simulink model "PC_Quadcopter_Simulation_Alchemist"  (R2023b)
settings: Solver=ode4  StartTime=0  StopTime=Tf  FixedStep=Ts  MaxStep=0.06  RelTol=1e-3  EnableMultiTasking=on
model workspace (MAT data in the model file):
  Sig = Simulink.Signal
  Sig.DataType = 'auto'
  Sig.Dimensions = -1
  Sig.DimensionsMode = 'auto'
  Sig.Complexity = 'auto'
  Sig.SampleTime = -1
  Sig.SamplingMode = 'auto'
values from neighbouring files (symbols this model uses):
  den_Pphi = conv(den_Qphi, num_Gphi)    [PC_Quadcopter_Alchemist_woDOBC.m]    (also in workingOcto.m)
  den_Ppsi = conv(den_Qpsi, num_Gpsi)    [PC_Quadcopter_Alchemist_woDOBC.m]    (also in workingOcto.m)
  den_Ptheta = conv(den_Qtheta, num_Gtheta)    [PC_Quadcopter_Alchemist_woDOBC.m]    (also in workingOcto.m)
  den_Px = conv(den_Qx, num_Gx)    [PC_Quadcopter_Alchemist_woDOBC.m]    (also in workingOcto.m)
  den_Py = conv(den_Qy, num_Gy)    [PC_Quadcopter_Alchemist_woDOBC.m]    (also in workingOcto.m)
  den_Pz = conv(den_Qz, num_Gz)    [PC_Quadcopter_Alchemist_woDOBC.m]    (also in workingOcto.m)
  Dist_Amp_phi = 0    [PC_Quadcopter_Alchemist_woDOBC.m]    (also in workingOcto.m)
  Dist_Amp_psi = 0    [PC_Quadcopter_Alchemist_woDOBC.m]    (also in workingOcto.m)
  Dist_Amp_theta = 0    [PC_Quadcopter_Alchemist_woDOBC.m]    (also in workingOcto.m)
  Dist_Amp_x = 0    [PC_Quadcopter_Alchemist_woDOBC.m]    (also in workingOcto.m)
  Dist_Amp_y = 0    [PC_Quadcopter_Alchemist_woDOBC.m]    (also in workingOcto.m)
  Dist_Amp_z = 0    [PC_Quadcopter_Alchemist_woDOBC.m]    (also in workingOcto.m)
  Dist_Freq_phi = 0    [PC_Quadcopter_Alchemist_woDOBC.m]    (also in workingOcto.m)
  Dist_Freq_psi = 0    [PC_Quadcopter_Alchemist_woDOBC.m]    (also in workingOcto.m)
  Dist_Freq_theta = 0    [PC_Quadcopter_Alchemist_woDOBC.m]    (also in workingOcto.m)
  Dist_Freq_x = 0    [PC_Quadcopter_Alchemist_woDOBC.m]    (also in workingOcto.m)
  Dist_Freq_y = 0    [PC_Quadcopter_Alchemist_woDOBC.m]    (also in workingOcto.m)
  Dist_Freq_z = 0    [PC_Quadcopter_Alchemist_woDOBC.m]    (also in workingOcto.m)
  Dist_mean_phi = 0    [PC_Quadcopter_Alchemist_woDOBC.m]    (also in workingOcto.m)
  Dist_mean_psi = 0    [PC_Quadcopter_Alchemist_woDOBC.m]    (also in workingOcto.m)
  Dist_mean_theta = 0    [PC_Quadcopter_Alchemist_woDOBC.m]    (also in workingOcto.m)
  Dist_mean_x = 0    [PC_Quadcopter_Alchemist_woDOBC.m]    (also in workingOcto.m)
  Dist_mean_y = 0    [PC_Quadcopter_Alchemist_woDOBC.m]    (also in workingOcto.m)
  Dist_mean_z = 0    [PC_Quadcopter_Alchemist_woDOBC.m]    (also in workingOcto.m)
  Dist_Var_phi = 0    [PC_Quadcopter_Alchemist_woDOBC.m]    (also in workingOcto.m)
  Dist_Var_psi = 0    [PC_Quadcopter_Alchemist_woDOBC.m]    (also in workingOcto.m)
  Dist_Var_theta = 0    [PC_Quadcopter_Alchemist_woDOBC.m]    (also in workingOcto.m)
  Dist_Var_x = 0    [PC_Quadcopter_Alchemist_woDOBC.m]    (also in workingOcto.m)
  Dist_Var_y = 0    [PC_Quadcopter_Alchemist_woDOBC.m]    (also in workingOcto.m)
  Dist_Var_z = 0    [PC_Quadcopter_Alchemist_woDOBC.m]    (also in workingOcto.m)
  DISTURBANCE = 0    [PC_Quadcopter_Alchemist_woDOBC.m]    (also in workingOcto.m)
  DOBC_phi = 0    [PC_Quadcopter_Alchemist_woDOBC.m]    (also in workingOcto.m)
  DOBC_psi = 0    [PC_Quadcopter_Alchemist_woDOBC.m]    (also in workingOcto.m)
  DOBC_theta = 0    [PC_Quadcopter_Alchemist_woDOBC.m]    (also in workingOcto.m)
  DOBC_x = 0    [PC_Quadcopter_Alchemist_woDOBC.m]    (also in workingOcto.m)
  DOBC_y = 0    [PC_Quadcopter_Alchemist_woDOBC.m]    (also in workingOcto.m)
  DOBC_z = 0    [PC_Quadcopter_Alchemist_woDOBC.m]    (also in workingOcto.m)
  GO = (sqrt((m*g)/(8*ct))-b)/cr    [PC_Quadcopter_Alchemist_woDOBC.m]    (also in workingOcto.m)
  IC =     [Hover_1m.mat]    (also in quadcopterDynamicsSFunction_Alchemist.m = block.DialogPrm(2).Data)
  INPUT_MODE_PHI = 0    [PC_Quadcopter_Alchemist_woDOBC.m]    (also in workingOcto.m)
  INPUT_MODE_THETA = 0    [PC_Quadcopter_Alchemist_woDOBC.m]    (also in workingOcto.m)
  INPUT_MODE_U = 0    [PC_Quadcopter_Alchemist_woDOBC.m]    (also in workingOcto.m)
  INPUT_MODE_V = 0    [PC_Quadcopter_Alchemist_woDOBC.m]    (also in workingOcto.m)
  Kd_phi = 2*Zc_phi*Wc_phi*Jx/Kphi    [PC_Quadcopter_Alchemist_woDOBC.m]    (also in workingOcto.m)
  Kd_psi = 2*Zc_psi*Wc_psi*Jz/Kpsi    [PC_Quadcopter_Alchemist_woDOBC.m]    (also in workingOcto.m)
  Kd_theta = 2*Zc_theta*Wc_theta*Jy/Ktheta    [PC_Quadcopter_Alchemist_woDOBC.m]    (also in workingOcto.m)
  Kd_u = Kp_u/50    [PC_Quadcopter_Alchemist_woDOBC.m]    (also in workingOcto.m)
  Kd_v = Kp_v/70    [PC_Quadcopter_Alchemist_woDOBC.m]    (also in workingOcto.m)
  Kd_x = Kp_x/5    (= 0.0710753921948)    [PC_Quadcopter_Alchemist_woDOBC.m]    (also in workingOcto.m = Kp_x/5)
  Kd_y = Kp_y/5    (= 0.014215078439)    [PC_Quadcopter_Alchemist_woDOBC.m]    (also in workingOcto.m = Kp_y/5)
  Kd_z = 2*Zc_z*Wc_z*m/Kz    [PC_Quadcopter_Alchemist_woDOBC.m]    (also in workingOcto.m = Kp_z/10)
  Ki_phi = Kp_phi/10    [PC_Quadcopter_Alchemist_woDOBC.m]    (also in workingOcto.m)
  Ki_psi = Kp_psi/20    [PC_Quadcopter_Alchemist_woDOBC.m]    (also in workingOcto.m)
  Ki_theta = Kp_theta/10    [PC_Quadcopter_Alchemist_woDOBC.m]    (also in workingOcto.m)
  Ki_u = Wc_u^2/g * 0.7    [PC_Quadcopter_Alchemist_woDOBC.m]    (also in workingOcto.m)
  Ki_v = Wc_v^2/g * 0.7    [PC_Quadcopter_Alchemist_woDOBC.m]    (also in workingOcto.m)
  Ki_x = Wc_x^2 * 0.7    (= 0.0442158277169)    [PC_Quadcopter_Alchemist_woDOBC.m]    (also in workingOcto.m = Wc_x^2 * 0.7)
  Ki_y = Wc_y^2 * 0.7    (= 0.00176863310868)    [PC_Quadcopter_Alchemist_woDOBC.m]    (also in workingOcto.m = Wc_y^2 * 0.7)
  Ki_z = 0    [PC_Quadcopter_Alchemist_woDOBC.m]    (also in workingOcto.m = Wc_z^2)
  Kp_phi = Wc_phi^2*Jx/Kphi    [PC_Quadcopter_Alchemist_woDOBC.m]    (also in workingOcto.m)
  Kp_psi = Wc_psi^2*Jz/Kpsi    [PC_Quadcopter_Alchemist_woDOBC.m]    (also in workingOcto.m)
  Kp_theta = Wc_theta^2*Jy/Ktheta    [PC_Quadcopter_Alchemist_woDOBC.m]    (also in workingOcto.m)
  Kp_u = 2*Zc_u*Wc_u/g    [PC_Quadcopter_Alchemist_woDOBC.m]    (also in workingOcto.m)
  Kp_v = 2*Zc_v*Wc_v/g    [PC_Quadcopter_Alchemist_woDOBC.m]    (also in workingOcto.m)
  Kp_x = 2*Wc_x*Zc_x    (= 0.355376960974)    [PC_Quadcopter_Alchemist_woDOBC.m]    (also in workingOcto.m = 2*Wc_x*Zc_x)
  Kp_y = 2*Wc_y*Zc_y    (= 0.0710753921948)    [PC_Quadcopter_Alchemist_woDOBC.m]    (also in workingOcto.m = 2*Wc_y*Zc_y)
  Kp_z = Wc_z^2*Jz/Kz    [PC_Quadcopter_Alchemist_woDOBC.m]    (also in workingOcto.m = 2*Wc_z*Zc_z)
  NOISE = 0    [PC_Quadcopter_Alchemist_woDOBC.m]    (also in workingOcto.m)
  num_Pphi = conv(num_Qphi, den_Gphi)    [PC_Quadcopter_Alchemist_woDOBC.m]    (also in workingOcto.m)
  num_Ppsi = conv(num_Qpsi, den_Gpsi)    [PC_Quadcopter_Alchemist_woDOBC.m]    (also in workingOcto.m)
  num_Ptheta = conv(num_Qtheta, den_Gtheta)    [PC_Quadcopter_Alchemist_woDOBC.m]    (also in workingOcto.m)
  num_Px = conv(num_Qx, den_Gx)    [PC_Quadcopter_Alchemist_woDOBC.m]    (also in workingOcto.m)
  num_Py = conv(num_Qy, den_Gy)    [PC_Quadcopter_Alchemist_woDOBC.m]    (also in workingOcto.m)
  num_Pz = conv(num_Qz, den_Gz)    [PC_Quadcopter_Alchemist_woDOBC.m]    (also in workingOcto.m)
  Phid = deg2rad(1)    [PC_Quadcopter_Alchemist_woDOBC.m]    (also in workingOcto.m = deg2rad(5))
  start_time = 5    [PC_Quadcopter_Alchemist_woDOBC.m]    (also in workingOcto.m = 1)
  step_0_ramp_1 = 0    [PC_Quadcopter_Alchemist_woDOBC.m]    (also in workingOcto.m)
  Thetad = deg2rad(1)    [PC_Quadcopter_Alchemist_woDOBC.m]    (also in workingOcto.m = deg2rad(0))
  Ts = 0.01    [PC_Quadcopter_Alchemist_woDOBC.m]    (also in workingOcto.m)
  Ud = 0    [PC_Quadcopter_Alchemist_woDOBC.m]    (also in workingOcto.m)
  Var_phi = 0.005^2    (= 2.5e-05)    [PC_Quadcopter_Alchemist_woDOBC.m]    (also in workingOcto.m)
  Var_psi = 0.005^2    (= 2.5e-05)    [PC_Quadcopter_Alchemist_woDOBC.m]    (also in workingOcto.m)
  Var_theta = 0.005^2    (= 2.5e-05)    [PC_Quadcopter_Alchemist_woDOBC.m]    (also in workingOcto.m)
  Var_u = 0.01^2    (= 0.0001)    [PC_Quadcopter_Alchemist_woDOBC.m]    (also in workingOcto.m)
  Var_v = 0.01^2    (= 0.0001)    [PC_Quadcopter_Alchemist_woDOBC.m]    (also in workingOcto.m)
  Var_w = 0.01^2    (= 0.0001)    [PC_Quadcopter_Alchemist_woDOBC.m]    (also in workingOcto.m)
  Var_x = 0.01^2    (= 0.0001)    [PC_Quadcopter_Alchemist_woDOBC.m]    (also in workingOcto.m)
  Var_y = 0.01^2    (= 0.0001)    [PC_Quadcopter_Alchemist_woDOBC.m]    (also in workingOcto.m)
  Var_z = 0.01^2    (= 0.0001)    [PC_Quadcopter_Alchemist_woDOBC.m]    (also in workingOcto.m)
  Vd = 0    [PC_Quadcopter_Alchemist_woDOBC.m]    (also in workingOcto.m)
  Vz = 0.1    [PC_Quadcopter_Alchemist_woDOBC.m]    (also in workingOcto.m)
  Xd = 0    [PC_Quadcopter_Alchemist_woDOBC.m]    (also in workingOcto.m = 1)
  Yd = 0    [PC_Quadcopter_Alchemist_woDOBC.m]    (also in workingOcto.m = 1)
  Zd = 2    [PC_Quadcopter_Alchemist_woDOBC.m]    (also in workingOcto.m = 1)
undefined symbols (not defined in the file or in its folder): den_Qphi, den_Qpsi, den_Qtheta, den_Qx, den_Qy, den_Qz, num_Qphi, num_Qpsi, num_Qtheta, num_Qx, num_Qy, num_Qz, quadModel
libraries: simulink x10, slpidlib x2, sharedtransform x1, uavutilslib x1
(part 1 of 2)
Description:
  | This is a configurable quadcopter simulation.
  | This Simulink model demonstates attitude control.
  | 
  | Additional quadcopter modeling and simulation materials available at:
  | github.com/dch33/Quad-Sim
  | 
  | Copyright (C) 2014 D. Hartman, K. Landis, S. Moreno, J. Kim, M. Mehrer
  | 
  | License:
  |     This program is free software: you can redistribute it and/or modify
  |     it under the terms of the GNU LESSER GENERAL PUBLIC LICENSE as published by
  |     the Free Software Foundation, either version 3 of the License, or
  |     (at your option) any later version.
  | 
  |     This program is distributed in the hope that it will be useful,
  |     but WITHOUT ANY WARRANTY; without even the implied warranty of
  |     MERCHANTABILITY or FITNESS FOR A PARTICULAR PURPOSE.  See the
  |     GNU General Public License for more details.
  | 
  |     You should have received a copy of the GNU LESSER GENERAL PUBLIC LICENSE
  |     along with this program.  If not, see <http://www.gnu.org/licenses/>.
settings Model: ModifiedComment=PC -- Fri Dec 18 19:27:23 2020 -- Version 5.370000e+00  Creator=David Hartman  LastModifiedBy=qkrrl
settings Model: ModifiedHistory=|
  | PC -- Fri Dec 18 19:27:23 2020 -- Version 5.370000e+00
  | 
  | PC -- Fri Dec 18 19:27:23 2020 -- Version 5.370000e+00
  | 
  | PC -- Fri Dec 18 18:41:02 2020 -- Version 5.360000e+00
  | 
  | PC -- Fri Dec 18 18:37:40 2020 -- Version 5.350000e+00
  | 
  | kangm -- Thu Dec 17 04:15:38 2020 -- Version 5.340000e+00
  | 
  | kangm -- Wed Dec 16 19:07:22 2020 -- Version 5.330000e+00
  | 
  | kangm -- Wed Dec 16 01:03:03 2020 -- Version 5.320000e+00
  | 
  | kangm -- Tue Dec 15 23:44:03 2020 -- Version 5.310000e+00
  | 
  | kangm -- Tue Dec 15 19:49:48 2020 -- Version 5.300000e+00
  | 
  | kangm -- Tue Dec 15 19:48:43 2020 -- Version 5.290000e+00
  | 
  | kangm -- Tue Dec 15 19:48:24 2020 -- Version 5.280000e+00
  | 
  | kangm -- Tue Dec 15 17:10:25 2020 -- Version 5.270000e+00
  | 
  | kangm -- Tue Dec 15 00:32:06 2020 -- Version 5.260000e+00
  | 
  | kangm -- Mon Dec 14 23:53:21 2020 -- Version 5.250000e+00
  | 
  | kangm -- Mon Dec 14 19:54:37 2020 -- Version 5.240000e+00
  | 
  | kangm -- Mon Dec 14 13:17:46 2020 -- Version 5.230000e+00
  | 
  | kangm -- Fri Dec 11 20:19:06 2020 -- Version 5.220000e+00
  | 
  | kangm -- Fri Dec 11 18:03:17 2020 -- Version 5.210000e+00
  | 
  | kangm -- Fri Dec 11 17:49:32 2020 -- Version 5.200000e+00
  | 
  | kangm -- Fri Dec 11 17:35:41 2020 -- Version 5.190000e+00
  | 
  | kangm -- Fri Dec 11 17:02:03 2020 -- Version 5.180000e+00
  | 
  | kangm -- Fri Dec 11 16:59:08 2020 -- Version 5.170000e+00
  | 
  | kangm -- Fri Dec 11 16:32:38 2020 -- Version 5.160000e+00
  | 
  | kangm -- Fri Dec 11 15:56:36 2020 -- Version 5.150000e+00
  | 
  | kangm -- Fri Dec 11 15:52:47 2020 -- Version 5.140000e+00
  | 
  | kangm -- Fri Dec 11 15:19:55 2020 -- Version 5.130000e+00
  | 
  | kangm -- Fri Dec 11 15:01:02 2020 -- Version 5.120000e+00
  | 
  | kangm -- Thu Dec 10 01:16:15 2020 -- Version 5.110000e+00
  | 
  | kangm -- Thu Dec 10 00:40:25 2020 -- Version 5.100000e+00
  | 
  | kangm -- Thu Dec 10 00:40:22 2020 -- Version 5.900000e+00
  | 
  | kangm -- Thu Dec 10 00:09:23 2020 -- Version 5.800000e+00
  | 
  | kangm -- Wed Dec 09 15:05:59 2020 -- Version 5.700000e+00
  | 
  | kangm -- Wed Dec 09 15:00:09 2020 -- Version 5.600000e+00
  | 
  | kangm -- Wed Dec 09 14:59:38 2020 -- Version 5.500000e+00
  | 
  | kangm -- Wed Dec 09 12:50:42 2020 -- Version 5.400000e+00
  | 
  | kangm -- Tue Dec 08 20:12:17 2020 -- Version 5.300000e+00
  | 
  | kangm -- Tue Dec 08 15:43:50 2020 -- Version 5.200000e+00
  | 
  | kangm -- Tue Dec 08 14:59:36 2020 -- Version 5.100000e+00
  | 
  | kangm -- Tue Dec 08 14:39:00 2020 -- Version 5
  | 
  | kangm -- Tue Dec 08 14:26:02 2020 -- Version 1.21
  | 
  | kangm -- Sat Dec 05 01:13:35 2020 -- Version 1.20
  | 
  | kangm -- Thu Dec 03 14:12:41 2020 -- Version 1.19
  | 
  | kangm -- Thu Dec 03 14:11:44 2020 -- Version 1.18
  | 
  | kangm -- Thu Dec 03 14:05:52 2020 -- Version 1.17
  | 
  | kangm -- Thu Nov 12 00:14:07 2020 -- Version 1.16
  | 
  | kangm -- Mon Nov 09 11:41:11 2020 -- Version 1.15
  | 
  | kangm -- Fri Nov 06 14:17:34 2020 -- Version 1.14
  | 
  | kangm -- Fri Nov 06 14:16:17 2020 -- Version 1.13
  | 
  | kangm -- Fri Nov 06 14:15:12 2020 -- Version 1.12
  | 
  | kangm -- Fri Nov 06 14:06:51 2020 -- Version 1.11
  | 
  | kangm -- Fri Nov 06 14:05:49 2020 -- Version 1.10
  | 
  | kangm -- Fri Nov 06 14:05:23 2020 -- Version 1.9
  | 
  | kangm -- Thu Nov 05 23:40:48 2020 -- Version 1.8
  | 
  | kangm -- Thu Nov 05 23:24:23 2020 -- Version 1.7
  | 
  | kangm -- Thu Nov 05 23:15:50 2020 -- Version 1.6
  | 
  | davidhartman -- Fri Jun 06 23:19:51 2014 -- Version 1.5
  | 
  | 
  | davidhartman -- Fri Jun 06 22:53:10 2014 -- Version 1.3
settings SolverCC: AlgebraicLoopSolver=TrustRegion  AutoInsertRateTranBlk=on
settings DataIOCC: SaveFormat=Array  SignalLogging=off  ReturnWorkspaceOutputs=off
settings OptimizationCC: DefaultParameterBehavior=Inlined  LifeSpan=inf
settings DebuggingCC: UnderspecifiedInitializationDetection=Classic  MergeDetectMultiDrivingBlocksExec=none  SolverPrmCheckMsg=warning  UnconnectedInputMsg=warning  UnconnectedOutputMsg=warning  UnconnectedLineMsg=warning  UniqueDataStoreMsg=warning  StateNameClashWarn=warning  StrictBusMsg=WarnOnBusTreatedAsVector  SFUnexpectedBacktrackingDiag=warning  SFNoUnconditionalDefaultTransitionDiag=warning  SFExecutionAtInitializationDiag=none  ArithmeticOperatorsInVariantConditions=warning
settings HardwareCC: ProdBitPerPointer=32  ProdBitPerSizeT=32  ProdBitPerPtrDiffT=32  ProdLargestAtomicFloat=None  ProdIntDivRoundTo=Undefined  ProdEndianess=Unspecified  ProdWordSize=32  ProdHWDeviceType=32-bit Generic
settings ModelReferenceCC: EnableRefExpFcnMdlSchedulingChecks=on  PropagateSignalLabelsOutOfModel=off
settings SFSimCC: SimUseLocalCustomCode=off  CustomCodeUndefinedFunction=UseInterfaceOnly
settings RTWCC: RTWUseLocalCustomCode=off  DLArmComputeVersion=19.05
settings CodeAppCC: StateflowObjectComments=on
settings GRTTargetCC: TargetLangStandard=C89/C90 (ANSI)
settings ConfigComp: CovMetricSettings=dw  CovSaveCumulativeToWorkspaceVar=on  CovSaveSingleToWorkspaceVar=on  CovExternalEMLEnable=off

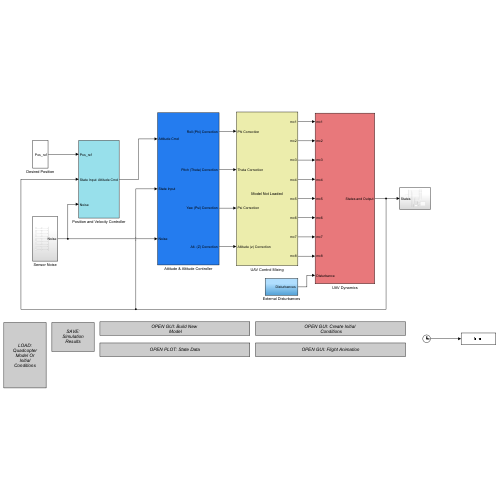
[thumbnail: Simulink's stored preview of the top-level diagram]
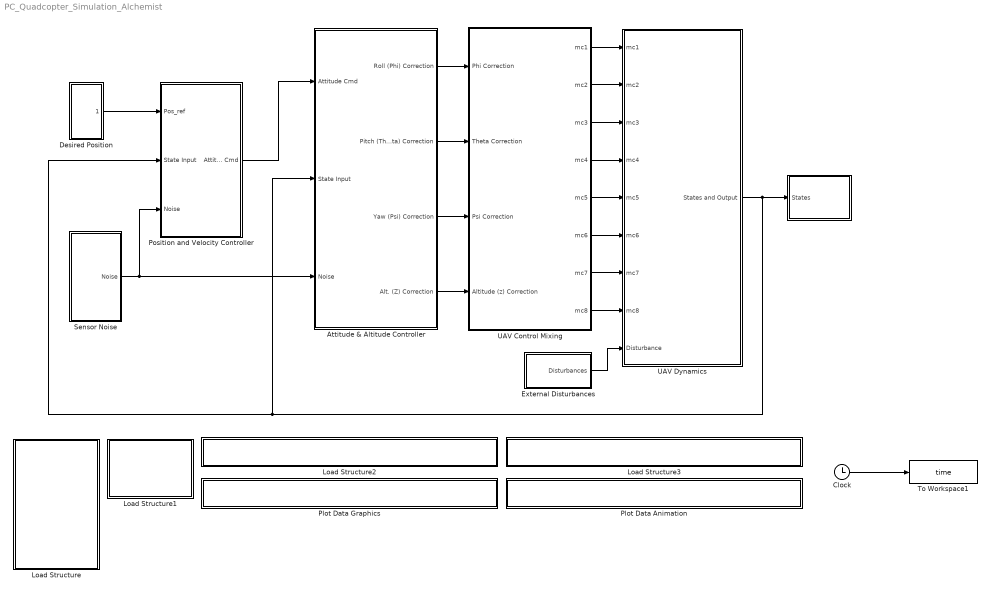
== system PC_Quadcopter_Simulation_Alchemist ==
  " " : Subsystem
  Attitude & Altitude Controller : Subsystem
  Clock : Clock
  Desired Position : Subsystem
  External Disturbances : Subsystem
  Load Structure : Subsystem
      settings: OpenFcn=|
      | uiopen('load')
      | if (exist('IC')==1 && exist('quadModel')==1)
      | set_param(bdroot, 'SimulationCommand', 'update')
      | end
      mask Display: fprintf('LOAD:\nQuadcopter\nModel Or\nInitial\nConditions');
  Load Structure1 : Subsystem
      settings: OpenFcn=|
      | if (exist('IC')==1 && exist('quadModel')==1 && exist('yout') && exist('tout'))
      | saveSimResults()
      | else
      | msgbox('No Data To Save!')
      | end
      mask Display: fprintf('SAVE:\nSimulation\nResults');
  Load Structure2 : Subsystem
      settings: OpenFcn=|
      | if exist('GUI_Modeling') == 2,
      | run('GUI_Modeling')
      | 
      | else
      | 
      | msgbox('The desired GUI must be first added to MATLABs path.')
      | 
      | end
      mask Display: fprintf('OPEN GUI: Build New \n Model');
  Load Structure3 : Subsystem
      settings: OpenFcn=|
      | if exist('GUI_IC') == 2,
      | run('GUI_IC')
      | 
      | else
      | 
      | msgbox('The desired GUI must be first added to MATLABs path.')
      | 
      | end
      mask Display: fprintf('OPEN GUI: Create Initial \n Conditions');
  Plot Data Animation : Subsystem
      settings: OpenFcn=|
      | if exist('QuadAnim4') == 2,
      |     if exist('yout')
      | 	run('QuadAnim4');
      |     else
      |     msgbox('Simulation must be run before data can be plotted.');
      |     end
      | else                                                                          msgbox('The desired GUI must be first added to MATLABs path.')
      | end
      mask Display: fprintf('OPEN GUI: Flight Animation')
  Plot Data Graphics : Subsystem
      settings: OpenFcn=|
      | if exist('yout')
      | yout = evalin('base', 'yout');
      | tout = evalin('base', 'tout');
      | quadPlots(yout, tout)
      | else
      | msgbox('Simulation must be run before data can be plotted.')
      | end
      mask Display: fprintf('OPEN PLOT: State Data')
  Position and Velocity Controller : Subsystem
  Sensor Noise : Subsystem
  To Workspace1 : ToWorkspace  VariableName=time  SampleTime=-1
      settings: Save2DSignal=2-D array (concatenate along first dimension)
  UAV Control Mixing : Subsystem
      mask Display:
      | modelLoaded = evalin('base','exist(''quadModel'',''var'')');
      | if (modelLoaded==1)
      |     if (evalin('base','quadModel.plusConfig'))
      |     fprintf([' \n' ' \n'  'Configuration "+"']);
      |     else if (~evalin('base','quadModel.plusConfig'))
      |         fprintf([' \n' ' \n' 'Configuration "X"']);
      |         end
      |     end
      | else
      |     fprintf([' \n' ' \n'  'Model Not Loaded']);
      | end
  UAV Dynamics : Subsystem
  wires:
  Attitude & Altitude Controller/1(Roll (Phi) Correction) -> UAV Control Mixing/1(Phi Correction)
  Attitude & Altitude Controller/2(Pitch (Theta) Correction) -> UAV Control Mixing/2(Theta Correction)
  Attitude & Altitude Controller/3(Yaw (Psi) Correction) -> UAV Control Mixing/3(Psi Correction)
  Attitude & Altitude Controller/4(Alt. (Z) Correction) -> UAV Control Mixing/4(Altitude (z) Correction)
  Position and Velocity Controller/1(Attitude Cmd) -> Attitude & Altitude Controller/1(Attitude Cmd)
  Clock/1 -> To Workspace1/1
  UAV Dynamics/1(States and Output) -> " "/1(States), Attitude & Altitude Controller/2(State Input), Position and Velocity Controller/2(State Input)
  Desired Position/1(Pos_ref) -> Position and Velocity Controller/1(Pos_ref)
  Sensor Noise/1(Noise) -> Position and Velocity Controller/3(Noise), Attitude & Altitude Controller/3(Noise)
  External Disturbances/1("Disturbances ") -> UAV Dynamics/9(Disturbance)
  UAV Control Mixing/1(mc1) -> UAV Dynamics/1(mc1)
  UAV Control Mixing/2(mc2) -> UAV Dynamics/2(mc2)
  UAV Control Mixing/3(mc3) -> UAV Dynamics/3(mc3)
  UAV Control Mixing/4(mc4) -> UAV Dynamics/4(mc4)
  UAV Control Mixing/5(mc5) -> UAV Dynamics/5(mc5)
  UAV Control Mixing/6(mc6) -> UAV Dynamics/6(mc6)
  UAV Control Mixing/7(mc7) -> UAV Dynamics/7(mc7)
  UAV Control Mixing/8(mc8) -> UAV Dynamics/8(mc8)

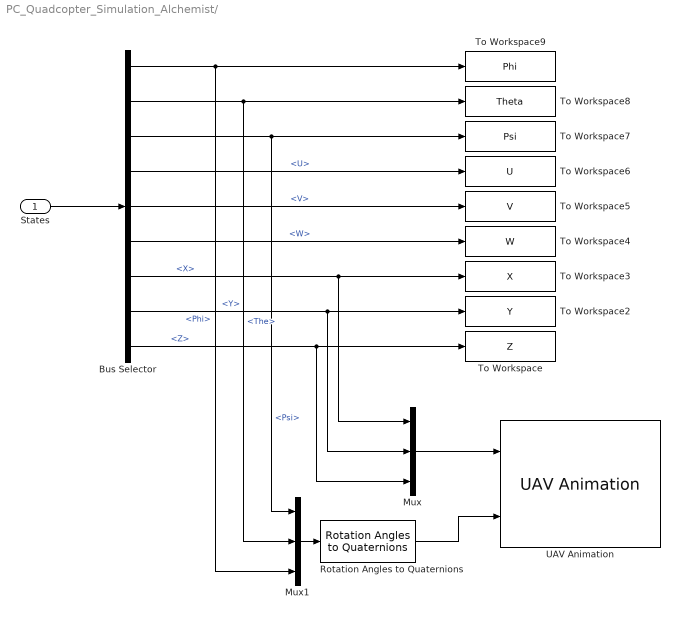
== system PC_Quadcopter_Simulation_Alchemist/  ==
  States : Inport
  Bus Selector : BusSelector  OutputSignals=Phi,The,Psi,U,V,W,X,Y,Z
  Mux : Mux  Inputs=3
  Mux1 : Mux  Inputs=3
  Rotation Angles to Quaternions : sharedtransform/Rotation Angles to Quaternions  rotationOrder=ZYX  aMode=aMode
  To Workspace : ToWorkspace  VariableName=Z  SampleTime=-1
      settings: Save2DSignal=2-D array (concatenate along first dimension)
  To Workspace2 : ToWorkspace  VariableName=Y  SampleTime=-1
      settings: Save2DSignal=2-D array (concatenate along first dimension)
  To Workspace3 : ToWorkspace  VariableName=X  SampleTime=-1
      settings: Save2DSignal=2-D array (concatenate along first dimension)
  To Workspace4 : ToWorkspace  VariableName=W  SampleTime=-1
      settings: Save2DSignal=2-D array (concatenate along first dimension)
  To Workspace5 : ToWorkspace  VariableName=V  SampleTime=-1
      settings: Save2DSignal=2-D array (concatenate along first dimension)
  To Workspace6 : ToWorkspace  VariableName=U  SampleTime=-1
      settings: Save2DSignal=2-D array (concatenate along first dimension)
  To Workspace7 : ToWorkspace  VariableName=Psi  SampleTime=-1
      settings: Save2DSignal=2-D array (concatenate along first dimension)
  To Workspace8 : ToWorkspace  VariableName=Theta  SampleTime=-1
      settings: Save2DSignal=2-D array (concatenate along first dimension)
  To Workspace9 : ToWorkspace  VariableName=Phi  SampleTime=-1
      settings: Save2DSignal=2-D array (concatenate along first dimension)
  UAV Animation : uavutilslib/UAV Animation  UAVType=Multirotor  UAVSize=1  InertialZDirection=Up  SampleTime=-1
  wires:
  Bus Selector/4 -> To Workspace6/1  "<U>"
  Bus Selector/5 -> To Workspace5/1  "<V>"
  Bus Selector/6 -> To Workspace4/1  "<W>"
  States/1 -> Bus Selector/1
  Bus Selector/2 -> Mux1/2, To Workspace8/1  "<The>"
  Bus Selector/1 -> Mux1/3, To Workspace9/1  "<Phi>"
  Bus Selector/9 -> Mux/3, To Workspace/1  "<Z>"
  Mux1/1 -> Rotation Angles to Quaternions/1
  Mux/1 -> UAV Animation/1
  Bus Selector/3 -> Mux1/1, To Workspace7/1  "<Psi>"
  Rotation Angles to Quaternions/1 -> UAV Animation/2
  Bus Selector/7 -> Mux/1, To Workspace3/1  "<X>"
  Bus Selector/8 -> Mux/2, To Workspace2/1  "<Y>"

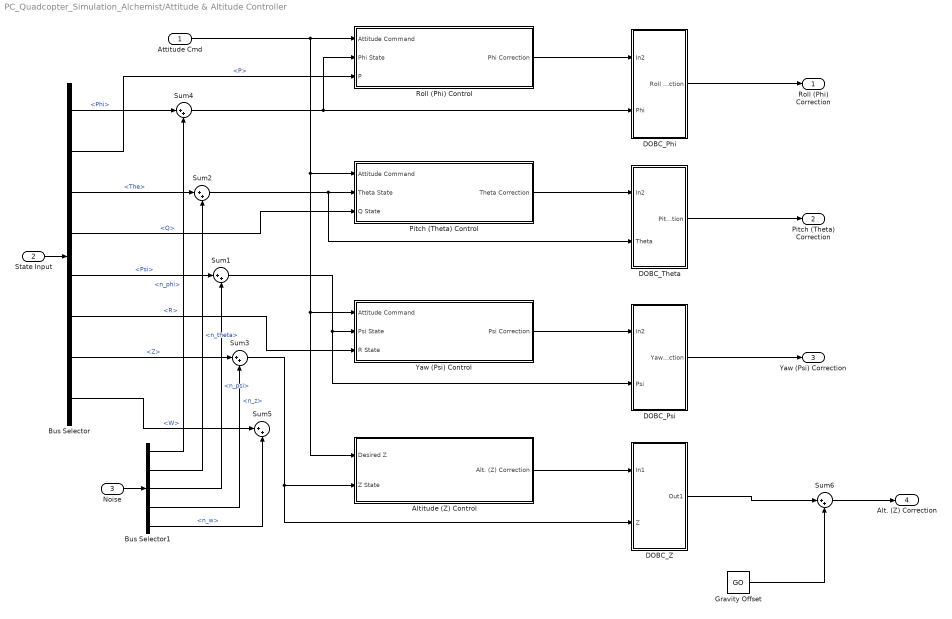
== system PC_Quadcopter_Simulation_Alchemist/Attitude & Altitude Controller ==
  Attitude Cmd : Inport
  State Input : Inport  Port=2
  Noise : Inport  Port=3
  Altitude (Z) Control : Subsystem  mask{Kpz=Kp_z, Kiz=Ki_z, Kdz=Kd_z, LimitOutput=on, USat=1, LSat=-1, GOffset=0}
      mask prompts: Kpz "Kp"; Kiz "Ki"; Kdz "Kd"; LimitOutput "Integral Saturation?"; USat "Upper saturation limit:"; LSat "Lower saturation limit:"; GOffset "Gravity Feedforward"
      mask help:
      | Adjust PID controller gains through this mask interface, or "look under mask" for more detailed adjustments.
      |
      | Note: Gravity Offset will not appear on block face as a value until simulation is run if it is the result of a formula involving the quadcopter model parameters.
      mask TypeOptions Kpz: Kpz/Gain
      mask TypeOptions Kiz: Kiz/Gain
      mask TypeOptions Kdz: Kdz/Gain
      mask TypeOptions LimitOutput:
      | Integrator
      | Limited/LimitOutput
      mask TypeOptions USat:
      | Integrator
      | Limited/UpperSaturationLimit
      mask TypeOptions LSat:
      | Integrator
      | Limited/LowerSaturationLimit
      mask TypeOptions GOffset: Gravity Offset (Level Flight)/Value
      mask Display:
      | fprintf(['Gravity Offset = ' num2str(GOffset) '\n' ...
      |     'Kp = ' num2str(Kpz) '\n' ...
      |     'Ki = ' num2str(Kiz) '\n' ...
      |     'Kd = ' num2str(Kdz) '\n' ...
      |     'Integral Saturation: ' LimitOutput]);
      | if strcmp(LimitOutput,'on')
      |     fprintf([' \n' ' \n' ' \n' ' \n' ' \n' '\n' ...
      |         'Limits: ' num2str(USat) ' to ' num2str(LSat)]);
      | end
  Bus Selector : BusSelector  OutputSignals=Phi,P,The,Q,Psi,R,Z,W
  Bus Selector1 : BusSelector  OutputSignals=n_phi,n_theta,n_psi,n_z,n_w
  DOBC_Phi : Subsystem
  DOBC_Psi : Subsystem
  DOBC_Theta : Subsystem
  DOBC_Z : Subsystem
  Gravity Offset : Constant  Value=GO
  Pitch (Theta) Control : Subsystem  mask{Kpt=Kp_theta, Kit=Ki_theta, Kdt=Kd_theta, LimitOutput=on, USat=1, LSat=-1}
      mask prompts: Kpt "Kp"; Kit "Ki"; Kdt "Kd"; LimitOutput "Integral Saturation?"; USat "Upper saturation limit:"; LSat "Lower saturation limit:"
      mask help: Adjust PID controller gains through this mask interface, or "look under mask" for more detailed adjustments.
      mask TypeOptions Kpt: Kpt/Gain
      mask TypeOptions Kit: Kit/Gain
      mask TypeOptions Kdt: Kdt/Gain
      mask TypeOptions LimitOutput:
      | Integrator
      | Limited/LimitOutput
      mask TypeOptions USat:
      | Integrator
      | Limited/UpperSaturationLimit
      mask TypeOptions LSat:
      | Integrator
      | Limited/LowerSaturationLimit
      mask Display:
      | fprintf(['Kp = ' num2str(Kpt) '\n' ...
      |     'Ki = ' num2str(Kit) '\n' ...
      |     'Kd = ' num2str(Kdt) '\n' ...
      |     'Integral Saturation: ' LimitOutput]);
      | if strcmp(LimitOutput,'on')
      |     fprintf([' \n' ' \n' ' \n' ' \n' '\n' ...
      |         'Limits: ' num2str(USat) ' to ' num2str(LSat)]);
      | end
  "Roll (Phi) Control " : Subsystem  mask{Kpp=Kp_phi, Kip=Ki_phi, Kdp=Kd_phi, LimitOutput=on, USat=1, LSat=-1}
      mask prompts: Kpp "Kp"; Kip "Ki"; Kdp "Kd"; LimitOutput "Integral Saturation:"; USat "Upper saturation limit:"; LSat "Lower saturation limit:"
      mask help:
      | Adjust PID controller gains through this mask interface, or "look under mask"
      | for more detailed adjustments.
      mask TypeOptions Kpp: Kpp/Gain
      mask TypeOptions Kip: Kip/Gain
      mask TypeOptions Kdp: Kdp/Gain
      mask TypeOptions LimitOutput:
      | Integrator
      | Limited/LimitOutput
      mask TypeOptions USat:
      | Integrator
      | Limited/UpperSaturationLimit
      mask TypeOptions LSat:
      | Integrator
      | Limited/LowerSaturationLimit
      mask Display:
      | fprintf(['Kp = ' num2str(Kpp) '\n' ...
      |     'Ki = ' num2str(Kip) '\n' ...
      |     'Kd = ' num2str(Kdp) '\n'...
      |     'Integral Saturation: ' LimitOutput]);
      | if strcmp(LimitOutput,'on')
      |     fprintf([' \n' ' \n' ' \n' ' \n' '\n' ...
      |         'Limits: ' num2str(USat) ' to ' num2str(LSat)]);
      | end
  Sum{1..6} (6 alike) : Sum  Inputs=|++
  Yaw (Psi) Control : Subsystem  mask{Kps=Kp_psi, Kis=Ki_psi, Kds=Kd_psi, LimitOutput=on, USat=1, LSat=-1}
      mask prompts: Kps "Kp"; Kis "Ki"; Kds "Kd"; LimitOutput "Integral Saturation?"; USat "Upper saturation limit:"; LSat "Lower saturation limit:"
      mask help: Adjust PID controller gains through this mask interface, or "look under mask" for more detailed adjustments.
      mask TypeOptions Kps: Kps/Gain
      mask TypeOptions Kis: Kit/Gain
      mask TypeOptions Kds: Kds/Gain
      mask TypeOptions LimitOutput:
      | Integrator
      | Limited/LimitOutput
      mask TypeOptions USat:
      | Integrator
      | Limited/UpperSaturationLimit
      mask TypeOptions LSat:
      | Integrator
      | Limited/LowerSaturationLimit
      mask Display:
      | fprintf(['Kp = ' num2str(Kps) '\n' ...
      |     'Ki = ' num2str(Kis) '\n' ...
      |     'Kd = ' num2str(Kds) '\n' ...
      |     'Integral Saturation: ' LimitOutput]);
      | if strcmp(LimitOutput,'on')
      |     fprintf([' \n' ' \n' ' \n' ' \n' '\n' ...
      |         'Limits: ' num2str(USat) ' to ' num2str(LSat)]);
      | end
  Roll (Phi) Correction : Outport  VectorParamsAs1DForOutWhenUnconnected=off
  Pitch (Theta) Correction : Outport  Port=2  VectorParamsAs1DForOutWhenUnconnected=off
  Yaw (Psi) Correction : Outport  Port=3  VectorParamsAs1DForOutWhenUnconnected=off
  Alt. (Z) Correction : Outport  Port=4  VectorParamsAs1DForOutWhenUnconnected=off
  wires:
  Bus Selector/6 -> Yaw (Psi) Control/3(R State)  "<R>"
  Bus Selector/4 -> Pitch (Theta) Control/3(Q State)  "<Q>"
  Bus Selector/2 -> "Roll (Phi) Control "/3(P)  "<P>"
  Attitude Cmd/1 -> Altitude (Z) Control/1(Desired Z), Yaw (Psi) Control/1(Attitude Command), Pitch (Theta) Control/1(Attitude Command), "Roll (Phi) Control "/1("Attitude Command ")
  State Input/1 -> Bus Selector/1
  Bus Selector/7 -> Sum3/1  "<Z>"
  Sum3/1 -> DOBC_Z/2(Z), Altitude (Z) Control/2(Z State)
  Altitude (Z) Control/1(Alt. (Z) Correction) -> DOBC_Z/1(In1)
  Yaw (Psi) Control/1(Psi Correction) -> DOBC_Psi/1(In2)
  Pitch (Theta) Control/1(Theta Correction) -> DOBC_Theta/1(In2)
  "Roll (Phi) Control "/1(Phi Correction) -> DOBC_Phi/1(In2)
  Bus Selector/5 -> Sum1/1  "<Psi>"
  Sum1/1 -> DOBC_Psi/2(Psi), Yaw (Psi) Control/2(Psi State)
  Bus Selector/3 -> Sum2/1  "<The>"
  Sum2/1 -> DOBC_Theta/2(Theta), Pitch (Theta) Control/2(Theta State)
  Sum4/1 -> "Roll (Phi) Control "/2(Phi State), DOBC_Phi/2(Phi)
  Bus Selector/1 -> Sum4/1  "<Phi>"
  Bus Selector1/2 -> Sum2/2  "<n_theta>"
  Bus Selector1/3 -> Sum1/2  "<n_psi>"
  Bus Selector1/4 -> Sum3/2  "<n_z>"
  Noise/1 -> Bus Selector1/1
  Bus Selector1/1 -> Sum4/2  "<n_phi>"
  Bus Selector/8 -> Sum5/1  "<W>"
  Bus Selector1/5 -> Sum5/2  "<n_w>"
  DOBC_Phi/1(Roll (Phi) Correction) -> Roll (Phi) Correction/1
  DOBC_Theta/1(Pitch (Theta) Correction) -> Pitch (Theta) Correction/1
  DOBC_Psi/1(Yaw (Psi) Correction) -> Yaw (Psi) Correction/1
  Sum6/1 -> Alt. (Z) Correction/1
  Gravity Offset/1 -> Sum6/2
  DOBC_Z/1(Out1) -> Sum6/1

== system PC_Quadcopter_Simulation_Alchemist/Desired Position ==
  Add : Sum  Inputs=+-+
  Bus Creator : BusCreator  Inputs=3
  Constant : Constant  Value=IC.Z
  Constant3 : Constant  Value=step_0_ramp_1
  Ramp1 : simulink/Sources/Ramp  slope=Vz  start=stop_time  InitialOutput=0
  Ramp4 : simulink/Sources/Ramp  slope=Vz  start=start_time  InitialOutput=0
  Step : Step  Time=start_time  Before=IC.Z  After=Zd  SampleTime=0
  Step1 : Step  Time=start_time  Before=IC.X  After=Xd  SampleTime=0
  Step2 : Step  Time=start_time  Before=IC.Y  After=Yd  SampleTime=0
  Switch : Switch  Criteria=u2 ~= 0  SaturateOnIntegerOverflow=off  InputSameDT=off
  To Workspace : ToWorkspace  VariableName=Zd_sim  SampleTime=-1
      settings: Save2DSignal=2-D array (concatenate along first dimension)
  To Workspace1 : ToWorkspace  VariableName=Yd_sim  SampleTime=-1
      settings: Save2DSignal=2-D array (concatenate along first dimension)
  To Workspace2 : ToWorkspace  VariableName=Xd_sim  SampleTime=-1
      settings: Save2DSignal=2-D array (concatenate along first dimension)
  Pos_ref : Outport
  wires:
  Step1/1 -> To Workspace2/1, Bus Creator/1  "X_cmd"
  Step2/1 -> To Workspace1/1, Bus Creator/2  "Y_cmd"
  Switch/1 -> Bus Creator/3, To Workspace/1  "Alt_cmd"
  Bus Creator/1 -> Pos_ref/1
  Add/1 -> Switch/1
  Constant3/1 -> Switch/2
  Ramp1/1 -> Add/3
  Constant/1 -> Add/1
  Ramp4/1 -> Add/2
  Step/1 -> Switch/3

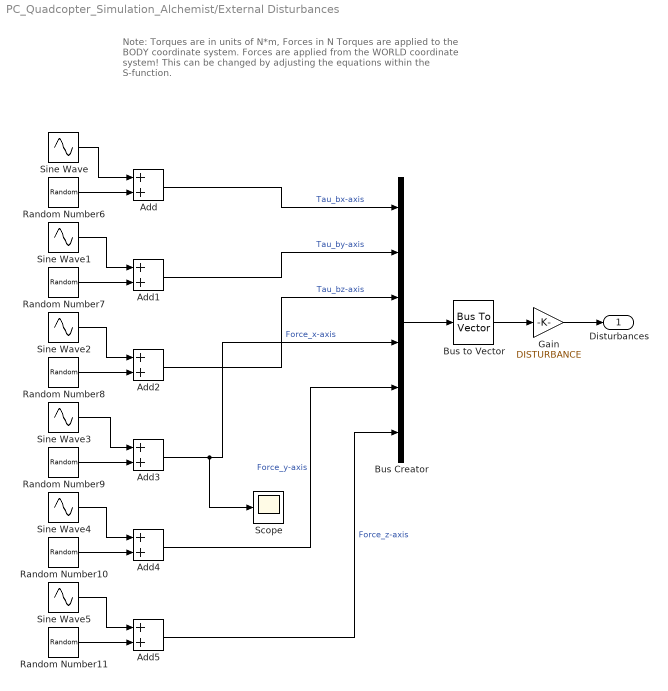
== system PC_Quadcopter_Simulation_Alchemist/External Disturbances ==
  note: Note: Torques are in units of N*m, Forces in N
      | Torques are applied to the BODY coordinate system.
      | Forces are applied from the WORLD coordinate system!
      | This can be changed by adjusting the equations within the S-function.
  Add{,1..5} (6 alike) : Sum
  Bus Creator : BusCreator  Inputs=6
  Bus to Vector : BusToVector
  Gain : Gain  Gain=DISTURBANCE
  Random Number10 : RandomNumber  Mean=Dist_mean_y  Variance=Dist_Var_y  Seed=453  SampleTime=Ts
  Random Number11 : RandomNumber  Mean=Dist_mean_z  Variance=Dist_Var_z  Seed=675  SampleTime=Ts
  Random Number6 : RandomNumber  Mean=Dist_mean_phi  Variance=Dist_Var_phi  Seed=324  SampleTime=Ts
  Random Number7 : RandomNumber  Mean=Dist_mean_theta  Variance=Dist_Var_theta  Seed=435  SampleTime=Ts
  Random Number8 : RandomNumber  Mean=Dist_mean_psi  Variance=Dist_Var_psi  Seed=764  SampleTime=Ts
  Random Number9 : RandomNumber  Mean=Dist_mean_x  Variance=Dist_Var_x  Seed=234  SampleTime=Ts
  Scope : Scope
  Sine Wave : Sin  Amplitude=Dist_Amp_phi  Frequency=Dist_Freq_phi  SampleTime=0
  Sine Wave1 : Sin  Amplitude=Dist_Amp_theta  Frequency=Dist_Freq_theta  SampleTime=0
  Sine Wave2 : Sin  Amplitude=Dist_Amp_psi  Frequency=Dist_Freq_psi  SampleTime=0
  Sine Wave3 : Sin  Amplitude=Dist_Amp_x  Frequency=Dist_Freq_x  SampleTime=0
  Sine Wave4 : Sin  Amplitude=Dist_Amp_y  Frequency=Dist_Freq_y  SampleTime=0
  Sine Wave5 : Sin  Amplitude=Dist_Amp_z  Frequency=Dist_Freq_z  SampleTime=0
  "Disturbances " : Outport  VectorParamsAs1DForOutWhenUnconnected=off
  wires:
  Bus Creator/1 -> Bus to Vector/1
  Bus to Vector/1 -> Gain/1
  Add4/1 -> Bus Creator/5  "Force_y-axis"
  Add3/1 -> Scope/1, Bus Creator/4  "Force_x-axis"
  Add2/1 -> Bus Creator/3  "Tau_bz-axis"
  Add1/1 -> Bus Creator/2  "Tau_by-axis"
  Add/1 -> Bus Creator/1  "Tau_bx-axis"
  Gain/1 -> "Disturbances "/1
  Add5/1 -> Bus Creator/6  "Force_z-axis"
  Sine Wave4/1 -> Add4/1
  Sine Wave5/1 -> Add5/1
  Sine Wave1/1 -> Add1/1
  Sine Wave2/1 -> Add2/1
  Random Number11/1 -> Add5/2
  Random Number6/1 -> Add/2
  Random Number7/1 -> Add1/2
  Random Number10/1 -> Add4/2
  Random Number8/1 -> Add2/2
  Sine Wave3/1 -> Add3/1
  Random Number9/1 -> Add3/2
  Sine Wave/1 -> Add/1

== system PC_Quadcopter_Simulation_Alchemist/Load Structure ==

== system PC_Quadcopter_Simulation_Alchemist/Load Structure1 ==

== system PC_Quadcopter_Simulation_Alchemist/Load Structure2 ==

== system PC_Quadcopter_Simulation_Alchemist/Load Structure3 ==

== system PC_Quadcopter_Simulation_Alchemist/Plot Data Animation ==

== system PC_Quadcopter_Simulation_Alchemist/Plot Data Graphics ==

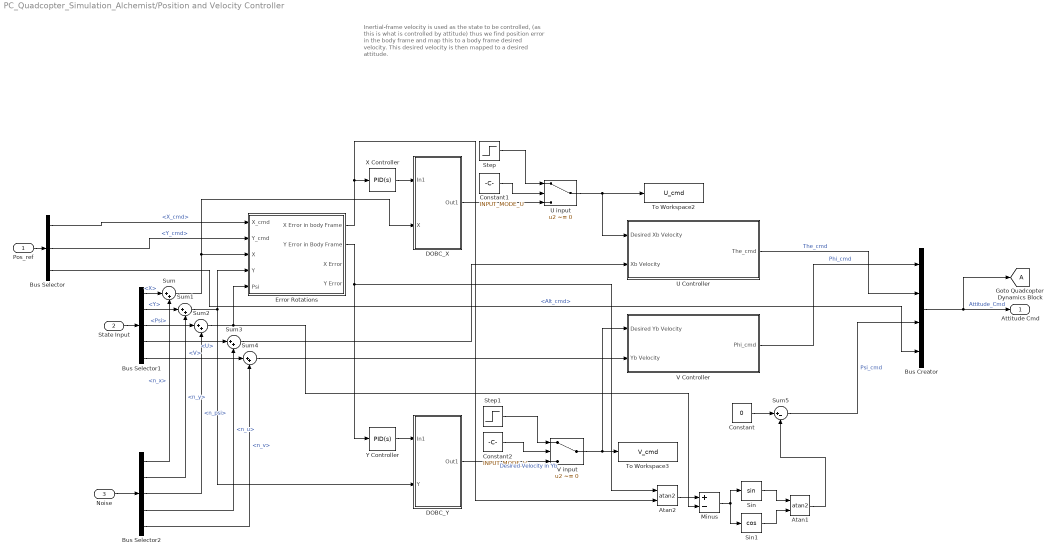
== system PC_Quadcopter_Simulation_Alchemist/Position and Velocity Controller ==
  note: Inertial-frame velocity is used as the state to be controlled,
      | (as this is what is controlled by attitude)
      | thus we find position error in the body frame
      | and map this to a body frame desired velocity. This desired
      | velocity is then mapped to a desired attitude.
  Pos_ref : Inport
  State Input : Inport  Port=2
  Noise : Inport  Port=3
  Atan1 : Trigonometry  Operator=atan2
  Atan2 : Trigonometry  Operator=atan2
  Bus Creator : BusCreator  Inputs=4
  Bus Selector : BusSelector  OutputSignals=X_cmd,Y_cmd,Alt_cmd
  Bus Selector1 : BusSelector  OutputSignals=X,Y,Psi,U,V
  Bus Selector2 : BusSelector  OutputSignals=n_x,n_y,n_psi,n_u,n_v
  Constant : Constant  Value=0
  Constant1 : Constant  Value=INPUT_MODE_U
  Constant2 : Constant  Value=INPUT_MODE_V
  DOBC_X : Subsystem
  DOBC_Y : Subsystem
  Error Rotations : Subsystem
  Goto Quadcopter Dynamics Block : Goto  TagVisibility=global
  Minus : Sum  Inputs=+-
  Sin : Trigonometry
  Sin1 : Trigonometry  Operator=cos
  Step : Step  Time=start_time  After=Ud  SampleTime=0
  Step1 : Step  Time=start_time  After=Vd  SampleTime=0
  Sum{,1..4} (5 alike) : Sum  Inputs=|++
  Sum5 : Sum  Inputs=|+-
  To Workspace2 : ToWorkspace  VariableName=U_cmd  SampleTime=-1
      settings: Save2DSignal=2-D array (concatenate along first dimension)
  To Workspace3 : ToWorkspace  VariableName=V_cmd  SampleTime=-1
      settings: Save2DSignal=2-D array (concatenate along first dimension)
  U Controller : Subsystem  mask{Kp=Kp_u, Kd=Kd_u, ASat=12*pi/180}
      mask prompts: Kp "Proportional Gain:"; Kd "Derivative Gain"; ASat "Attitude Limit (+/- radians):"
      mask TypeOptions Kp: Kpt/Gain
      mask TypeOptions Kd: Kdt/Gain
      mask TypeOptions ASat: Attitude Limits_Theta/UpperLimit
      mask Display:
      | fprintf(['Kp = ' num2str(Kp) '\n' ...
      |     'Kd = ' num2str(Kd) '\n' ...
      |     'Attitude Limit (+/-): ' num2str(ASat*180/pi) '°']);
  U input : Switch  Criteria=u2 ~= 0  SaturateOnIntegerOverflow=off  InputSameDT=off
  V Controller : Subsystem  mask{Kp=Kp_v, Kd=Kd_v, ASat=12*pi/180}
      mask prompts: Kp "Proportional Gain"; Kd "Derivative Gain"; ASat "Attitude Limit (+/- radians):"
      mask TypeOptions Kp: Kpp/Gain
      mask TypeOptions Kd: Kdp/Gain
      mask TypeOptions ASat: Attitude Limits_Phi/UpperLimit
      mask Display:
      | fprintf(['Kp = ' num2str(Kp) '\n' ...
      |     'Kd = ' num2str(Kd) '\n' ...
      |     'Attitude Limit (+/-): ' num2str(ASat*180/pi) '°']);
  V input : Switch  Criteria=u2 ~= 0  SaturateOnIntegerOverflow=off  InputSameDT=off
  X Controller : slpidlib/PID Controller  Controller=PID  Form=Parallel  TimeDomain=Continuous-time  UseExternalTs=off  SampleTime=-1  IntegratorMethod=Forward Euler  FilterMethod=Forward Euler  ControllerParametersSource=internal  P=Kp_x  I=Ki_x  UseKiTs=off  D=Kd_x  N=100  UseFilter=on  TunerSelectOption=Transfer Function Based (PID Tuner App)  InitialConditionSource=internal  InitialConditionForIntegrator=0  InitialConditionForFilter=0  DifferentiatorICPrevScaledInput=0  ExternalReset=none  TrackingMode=off  Kt=1  LimitOutput=off  SatLimitsSource=internal  UpperSaturationLimit=inf  LowerSaturationLimit=-inf  LinearizeAsGain=on  AntiWindupMode=none  Kb=1  LimitIntegrator=off  UpperIntegratorSaturationLimit=inf  LowerIntegratorSaturationLimit=-inf  POutMin=[]  POutMax=[]  IOutMin=[]  IOutMax=[]  DOutMin=[]  DOutMax=[]  NOutMin=[]  NOutMax=[]  SumOutMin=[]  SumOutMax=[]  SaturationOutMin=[]  SaturationOutMax=[]  PParamMin=[]  PParamMax=[]  IParamMin=[]  IParamMax=[]  DParamMin=[]  DParamMax=[]  NParamMin=[]  NParamMax=[]  KbParamMin=[]  KbParamMax=[]  KtParamMin=[]  KtParamMax=[]  KbOutMin=[]  KbOutMax=[]  KtOutMin=[]  KtOutMax=[]  IntegratorOutMin=[]  IntegratorOutMax=[]  FilterOutMin=[]  FilterOutMax=[]  SumI1OutMin=[]  SumI1OutMax=[]  SumI2OutMin=[]  SumI2OutMax=[]  SumI3OutMin=[]  SumI3OutMax=[]  SumI4OutMin=[]  SumI4OutMax=[]  SumDOutMin=[]  SumDOutMax=[]  DifferentiatorOutMin=[]  DifferentiatorOutMax=[]  FilterDiffOutCoefMin=[]  FilterDiffOutCoefMax=[]  ReciprocalOutMin=[]  ReciprocalOutMax=[]  SumDenOutMin=[]  SumDenOutMax=[]  SumNumOutMin=[]  SumNumOutMax=[]  DivideOutMin=[]  DivideOutMax=[]  UdiffTsProdOutMin=[]  UdiffTsProdOutMax=[]  NTsProdOutMin=[]  NTsProdOutMax=[]  UintegralTsProdOutMin=[]  UintegralTsProdOutMax=[]  UngainTsProdOutMin=[]  UngainTsProdOutMax=[]  ClampingZeroOutDataTypeStr=Inherit: Inherit via back propagation  ClampingZeroOutMin=[]  ClampingZeroOutMax=[]  FilterDenConstantOutDataTypeStr=Inherit: Inherit via back propagation  FilterDenConstantOutMin=[]  FilterDenConstantOutMax=[]  PCopyOutDataTypeStr=Inherit: Inherit via back propagation  PCopyOutMin=[]  PCopyOutMax=[]  NCopyOutDataTypeStr=Inherit: Inherit via back propagation  NCopyOutMin=[]  NCopyOutMax=[]  IntegratorContinuousStateAttributes=''  IntegratorStateMustResolveToSignalObject=off  IntegratorRTWStateStorageClass=Auto  FilterContinuousStateAttributes=''  FilterStateMustResolveToSignalObject=off  FilterRTWStateStorageClass=Auto  ParallelPVariant=InternalParameters  IdealPVariant=Disabled  IVariant=InternalParameters  DVariant=InternalParameters  IntegratorVariant=Continuous  SatVariant=Disabled  AWVariant=Passthrough  PCopyVariant=Disabled  TRVariant=Disabled  FdbkBlocksVariant=Forward  IdealPFdbkVariant=Disabled  SatFdbkVariant=Disabled  DerivativeFilterVariant=ContFilter  NVariant=InternalParameters  NCopyVariant=Disabled  FilterICVariant=InternalICsFilter  IntegratorICVariant=InternalICs  ExternalResetVariant=Disabled  TRSumVariant=Passthrough  SumFdbkVariant=Disabled  SumVariant=Sum_PID  TsampFilterVariant=InternalTs  TsampNgainVariant=Passthrough  TsampIntegralVariant=Disabled_SignalSpec  ExternalSaturationOutDataTypeStr=Inherit: Same as second input
  Y Controller : slpidlib/PID Controller  Controller=PID  Form=Parallel  TimeDomain=Continuous-time  UseExternalTs=off  SampleTime=-1  IntegratorMethod=Forward Euler  FilterMethod=Forward Euler  ControllerParametersSource=internal  P=Kp_y  I=Ki_y  UseKiTs=off  D=Kd_y  N=100  UseFilter=on  TunerSelectOption=Transfer Function Based (PID Tuner App)  InitialConditionSource=internal  InitialConditionForIntegrator=0  InitialConditionForFilter=0  DifferentiatorICPrevScaledInput=0  ExternalReset=none  TrackingMode=off  Kt=1  LimitOutput=off  SatLimitsSource=internal  UpperSaturationLimit=inf  LowerSaturationLimit=-inf  LinearizeAsGain=on  AntiWindupMode=none  Kb=1  LimitIntegrator=off  UpperIntegratorSaturationLimit=inf  LowerIntegratorSaturationLimit=-inf  POutMin=[]  POutMax=[]  IOutMin=[]  IOutMax=[]  DOutMin=[]  DOutMax=[]  NOutMin=[]  NOutMax=[]  SumOutMin=[]  SumOutMax=[]  SaturationOutMin=[]  SaturationOutMax=[]  PParamMin=[]  PParamMax=[]  IParamMin=[]  IParamMax=[]  DParamMin=[]  DParamMax=[]  NParamMin=[]  NParamMax=[]  KbParamMin=[]  KbParamMax=[]  KtParamMin=[]  KtParamMax=[]  KbOutMin=[]  KbOutMax=[]  KtOutMin=[]  KtOutMax=[]  IntegratorOutMin=[]  IntegratorOutMax=[]  FilterOutMin=[]  FilterOutMax=[]  SumI1OutMin=[]  SumI1OutMax=[]  SumI2OutMin=[]  SumI2OutMax=[]  SumI3OutMin=[]  SumI3OutMax=[]  SumI4OutMin=[]  SumI4OutMax=[]  SumDOutMin=[]  SumDOutMax=[]  DifferentiatorOutMin=[]  DifferentiatorOutMax=[]  FilterDiffOutCoefMin=[]  FilterDiffOutCoefMax=[]  ReciprocalOutMin=[]  ReciprocalOutMax=[]  SumDenOutMin=[]  SumDenOutMax=[]  SumNumOutMin=[]  SumNumOutMax=[]  DivideOutMin=[]  DivideOutMax=[]  UdiffTsProdOutMin=[]  UdiffTsProdOutMax=[]  NTsProdOutMin=[]  NTsProdOutMax=[]  UintegralTsProdOutMin=[]  UintegralTsProdOutMax=[]  UngainTsProdOutMin=[]  UngainTsProdOutMax=[]  ClampingZeroOutDataTypeStr=Inherit: Inherit via back propagation  ClampingZeroOutMin=[]  ClampingZeroOutMax=[]  FilterDenConstantOutDataTypeStr=Inherit: Inherit via back propagation  FilterDenConstantOutMin=[]  FilterDenConstantOutMax=[]  PCopyOutDataTypeStr=Inherit: Inherit via back propagation  PCopyOutMin=[]  PCopyOutMax=[]  NCopyOutDataTypeStr=Inherit: Inherit via back propagation  NCopyOutMin=[]  NCopyOutMax=[]  IntegratorContinuousStateAttributes=''  IntegratorStateMustResolveToSignalObject=off  IntegratorRTWStateStorageClass=Auto  FilterContinuousStateAttributes=''  FilterStateMustResolveToSignalObject=off  FilterRTWStateStorageClass=Auto  ParallelPVariant=InternalParameters  IdealPVariant=Disabled  IVariant=InternalParameters  DVariant=InternalParameters  IntegratorVariant=Continuous  SatVariant=Disabled  AWVariant=Passthrough  PCopyVariant=Disabled  TRVariant=Disabled  FdbkBlocksVariant=Forward  IdealPFdbkVariant=Disabled  SatFdbkVariant=Disabled  DerivativeFilterVariant=ContFilter  NVariant=InternalParameters  NCopyVariant=Disabled  FilterICVariant=InternalICsFilter  IntegratorICVariant=InternalICs  ExternalResetVariant=Disabled  TRSumVariant=Passthrough  SumFdbkVariant=Disabled  SumVariant=Sum_PID  TsampFilterVariant=InternalTs  TsampNgainVariant=Passthrough  TsampIntegralVariant=Disabled_SignalSpec  ExternalSaturationOutDataTypeStr=Inherit: Same as second input
  Attitude Cmd : Outport
  wires:
  State Input/1 -> Bus Selector1/1
  Pos_ref/1 -> Bus Selector/1
  Bus Selector/3 -> Bus Creator/4  "<Alt_cmd>"
  Bus Creator/1 -> Attitude Cmd/1, Goto Quadcopter Dynamics Block/1  "Attitude_Cmd"
  Bus Selector/1 -> Error Rotations/1(X_cmd)  "<X_cmd>"
  Bus Selector/2 -> Error Rotations/2(Y_cmd)  "<Y_cmd>"
  Error Rotations/1(X Error in body Frame) -> Atan2/2, X Controller/1
  Noise/1 -> Bus Selector2/1
  Bus Selector1/1 -> Sum/1  "<X>"
  Sum/1 -> DOBC_X/2(X), Error Rotations/3(X)
  Bus Selector2/1 -> Sum/2  "<n_x>"
  Bus Selector1/2 -> Sum1/1  "<Y>"
  Sum1/1 -> DOBC_Y/2(Y), Error Rotations/4(Y)
  Bus Selector2/2 -> Sum1/2  "<n_y>"
  Bus Selector1/3 -> Sum2/1  "<Psi>"
  Sum2/1 -> Minus/2, Error Rotations/5(Psi)
  Bus Selector2/3 -> Sum2/2  "<n_psi>"
  Bus Selector1/4 -> Sum3/1  "<U>"
  Sum3/1 -> U Controller/2(Xb Velocity)
  Bus Selector2/4 -> Sum3/2  "<n_u>"
  Bus Selector1/5 -> Sum4/1  "<V>"
  Sum4/1 -> V Controller/2(Yb Velocity)
  Bus Selector2/5 -> Sum4/2  "<n_v>"
  Error Rotations/2(Y Error in Body Frame) -> Atan2/1, Y Controller/1
  X Controller/1 -> DOBC_X/1(In1)
  Y Controller/1 -> DOBC_Y/1(In1)
  DOBC_X/1(Out1) -> U input/3
  Constant1/1 -> U input/2
  Step/1 -> U input/1
  U input/1 -> To Workspace2/1, U Controller/1(Desired Xb Velocity)
  Constant2/1 -> V input/2
  Step1/1 -> V input/1
  DOBC_Y/1(Out1) -> V input/3  "Desired Velocity in Yb"
  V input/1 -> V Controller/1(Desired Yb Velocity), To Workspace3/1
  U Controller/1(The_cmd) -> Bus Creator/2  "The_cmd"
  V Controller/1(Phi_cmd) -> Bus Creator/1  "Phi_cmd"
  Sum5/1 -> Bus Creator/3  "Psi_cmd"
  Constant/1 -> Sum5/1
  Atan2/1 -> Minus/1
  Sin/1 -> Atan1/1
  Sin1/1 -> Atan1/2
  Minus/1 -> Sin1/1, Sin/1
  Atan1/1 -> Sum5/2

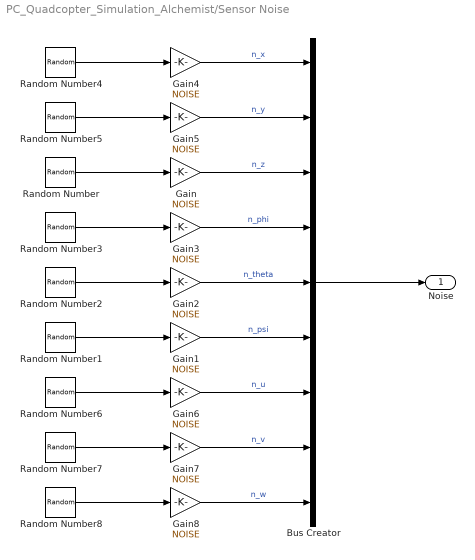
== system PC_Quadcopter_Simulation_Alchemist/Sensor Noise ==
  Bus Creator : BusCreator  Inputs=9
  Gain{,1..8} (9 alike) : Gain  Gain=NOISE
  Random Number : RandomNumber  Variance=Var_z  Seed=3214  SampleTime=Ts
  Random Number1 : RandomNumber  Variance=Var_psi  Seed=42529  SampleTime=Ts
  Random Number2 : RandomNumber  Variance=Var_theta  Seed=32456  SampleTime=Ts
  Random Number3 : RandomNumber  Variance=Var_phi  Seed=5664  SampleTime=Ts
  Random Number4 : RandomNumber  Variance=Var_x  Seed=4542  SampleTime=Ts
  Random Number5 : RandomNumber  Variance=Var_y  Seed=5345232  SampleTime=Ts
  Random Number6 : RandomNumber  Variance=Var_u  Seed=4252923  SampleTime=Ts
  Random Number7 : RandomNumber  Variance=Var_v  Seed=324633  SampleTime=Ts
  Random Number8 : RandomNumber  Variance=Var_w  Seed=324633  SampleTime=Ts
  Noise : Outport
  wires:
  Random Number/1 -> Gain/1
  Random Number1/1 -> Gain1/1
  Random Number3/1 -> Gain3/1
  Random Number2/1 -> Gain2/1
  Gain/1 -> Bus Creator/3  "n_z"
  Gain1/1 -> Bus Creator/6  "n_psi"
  Gain2/1 -> Bus Creator/5  "n_theta"
  Gain3/1 -> Bus Creator/4  "n_phi"
  Gain4/1 -> Bus Creator/1  "n_x"
  Random Number4/1 -> Gain4/1
  Random Number5/1 -> Gain5/1
  Gain5/1 -> Bus Creator/2  "n_y"
  Bus Creator/1 -> Noise/1
  Gain6/1 -> Bus Creator/7  "n_u"
  Random Number6/1 -> Gain6/1
  Random Number7/1 -> Gain7/1
  Gain7/1 -> Bus Creator/8  "n_v"
  Random Number8/1 -> Gain8/1
  Gain8/1 -> Bus Creator/9  "n_w"

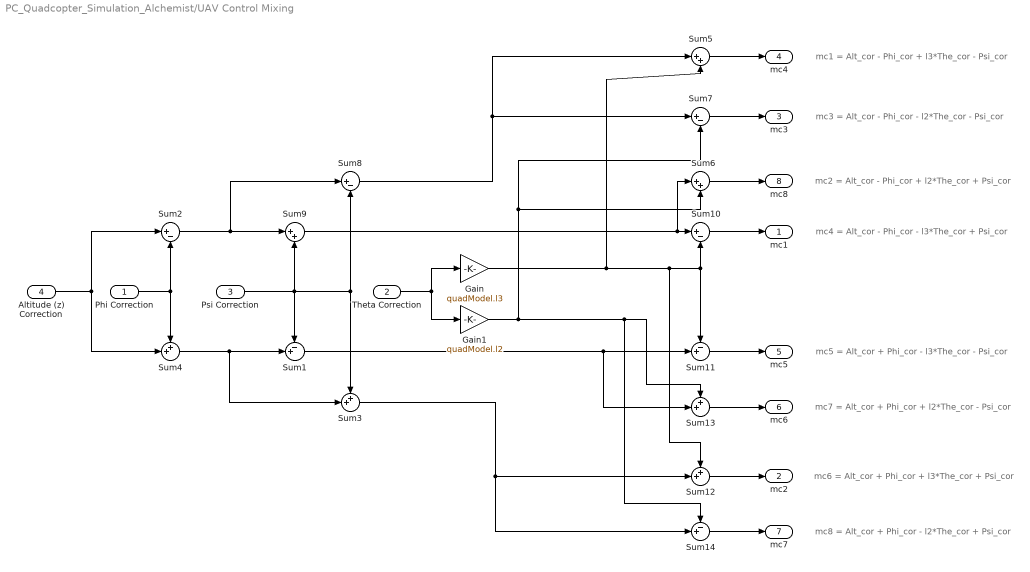
== system PC_Quadcopter_Simulation_Alchemist/UAV Control Mixing ==
  note: mc1 = Alt_cor - Phi_cor + l3*The_cor - Psi_cor
  note: mc2 = Alt_cor - Phi_cor + l2*The_cor + Psi_cor
  note: mc3 = Alt_cor - Phi_cor - l2*The_cor - Psi_cor
  note: mc4 = Alt_cor - Phi_cor - l3*The_cor + Psi_cor
  note: mc5 = Alt_cor + Phi_cor - l3*The_cor - Psi_cor
  note: mc6 = Alt_cor + Phi_cor + l3*The_cor + Psi_cor
  note: mc7 = Alt_cor + Phi_cor + l2*The_cor - Psi_cor
  note: mc8 = Alt_cor + Phi_cor - l2*The_cor + Psi_cor
  Phi Correction : Inport
  Theta Correction : Inport  Port=2
  Psi Correction : Inport  Port=3
  Altitude (z) Correction : Inport  Port=4
  Gain : Gain  Gain=quadModel.l3
  Gain1 : Gain  Gain=quadModel.l2
  Sum1 : Sum  Inputs=-+|
  Sum{2,7..8,10} (4 alike) : Sum  Inputs=|+-
  Sum11 : Sum  Inputs=-+|
  Sum{3..4,12..13} (4 alike) : Sum  Inputs=++|
  Sum14 : Sum  Inputs=-+|
  Sum5 : Sum  Inputs=|++
  Sum6 : Sum  Inputs=|++
  Sum9 : Sum  Inputs=|++
  mc1 : Outport  VectorParamsAs1DForOutWhenUnconnected=off
  mc2 : Outport  Port=2  VectorParamsAs1DForOutWhenUnconnected=off
  mc3 : Outport  Port=3  VectorParamsAs1DForOutWhenUnconnected=off
  mc4 : Outport  Port=4  VectorParamsAs1DForOutWhenUnconnected=off
  mc5 : Outport  Port=5  VectorParamsAs1DForOutWhenUnconnected=off
  mc6 : Outport  Port=6  VectorParamsAs1DForOutWhenUnconnected=off
  mc7 : Outport  Port=7  VectorParamsAs1DForOutWhenUnconnected=off
  mc8 : Outport  Port=8  VectorParamsAs1DForOutWhenUnconnected=off
  wires:
  Sum4/1 -> Sum3/2, Sum1/2
  Phi Correction/1 -> Sum2/2, Sum4/1
  Psi Correction/1 -> Sum9/2, Sum8/2, Sum3/1, Sum1/1
  Altitude (z) Correction/1 -> Sum4/2, Sum2/1
  Sum2/1 -> Sum8/1, Sum9/1
  Theta Correction/1 -> Gain1/1, Gain/1
  Sum8/1 -> Sum5/1, Sum7/1
  Gain/1 -> Sum12/1, Sum11/1, Sum10/2, Sum5/2
  Sum5/1 -> mc4/1
  Gain1/1 -> Sum13/1, Sum14/1, Sum6/2, Sum7/2
  Sum6/1 -> mc8/1
  Sum9/1 -> Sum6/1, Sum10/1
  Sum7/1 -> mc3/1
  Sum10/1 -> mc1/1
  Sum11/1 -> mc5/1
  Sum12/1 -> mc2/1
  Sum13/1 -> mc6/1
  Sum14/1 -> mc7/1
  Sum1/1 -> Sum13/2, Sum11/2
  Sum3/1 -> Sum14/2, Sum12/2
